simulink model "liner_vs_uliner"  (R2023b)
settings: Solver=VariableStepAuto  StartTime=0.0  StopTime=5  RelTol=1e-9
values from neighbouring files (symbols this model uses):
  A = [A_x, A_y, A_z, A_phi, A_thetha, A_psi]    [Overforingsfunksjon_Translasjon.m]
  Cd = 1.5    [Overforingsfunksjon_Translasjon.m]
  D_jag = [M(1),rho_vann*Cd*A_x*X_2]    [Overforingsfunksjon_Translasjon.m]
  M = M_rb + M_A    [Overforingsfunksjon_Translasjon.m]
  rho_vann = 1000    [Overforingsfunksjon_Translasjon.m]
settings Model: Creator=anneb  LastModifiedBy=anneb

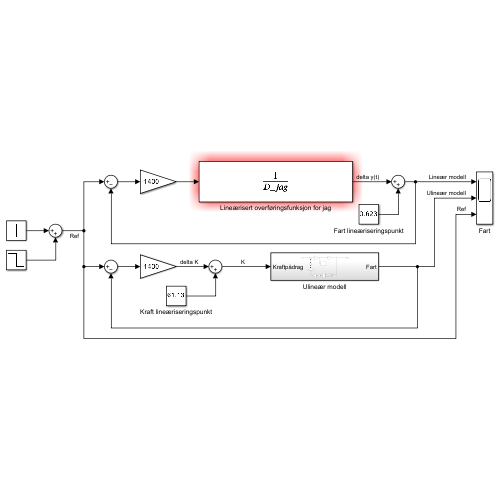
[thumbnail: Simulink's stored preview of the top-level diagram]
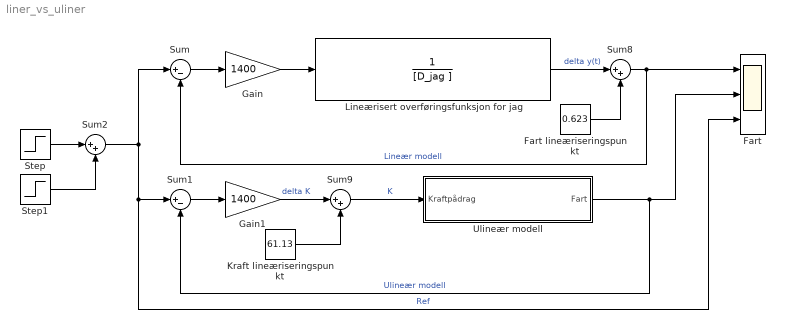
== system liner_vs_uliner ==
  Fart : Scope  NumInputPorts=3
  Fart lineæriseringspunkt : Constant  Value=0.623
  Gain : Gain  Gain=1400
  Gain1 : Gain  Gain=1400
  Kraft lineæriseringspunkt : Constant  Value=61.13
  Lineærisert overføringsfunksjon for jag : TransferFcn  Denominator=[D_jag ]
  Step : Step  Before=0.623  After=0.89  SampleTime=0
  Step1 : Step  Time=3  After=-0.89  SampleTime=0
  Sum : Sum  Inputs=|+-
  Sum1 : Sum  Inputs=|+-
  Sum2 : Sum  Inputs=|++
  Sum8 : Sum  Inputs=|++
  Sum9 : Sum  Inputs=|++
  Ulineær modell : Subsystem
  wires:
  Lineærisert overføringsfunksjon for jag/1 -> Sum8/1  "delta y(t)"
  Sum8/1 -> Sum/2, Fart/1  "Lineær modell"
  Ulineær modell/1(Fart) -> Sum1/2, Fart/2  "Ulineær modell"
  Step/1 -> Sum2/1
  Fart lineæriseringspunkt/1 -> Sum8/2
  Kraft lineæriseringspunkt/1 -> Sum9/2
  Sum9/1 -> Ulineær modell/1(Kraftpådrag)  "K"
  Gain/1 -> Lineærisert overføringsfunksjon for jag/1
  Gain1/1 -> Sum9/1  "delta K"
  Sum/1 -> Gain/1
  Sum1/1 -> Gain1/1
  Step1/1 -> Sum2/2
  Sum2/1 -> Sum1/1, Fart/3, Sum/1  "Ref"

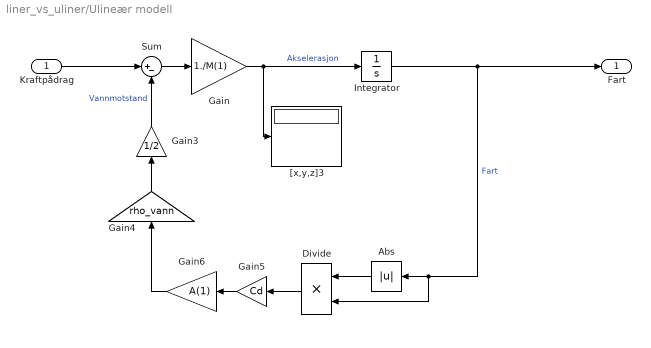
== system liner_vs_uliner/Ulineær modell ==
  Kraftpådrag : Inport
  Abs : Abs  SaturateOnIntegerOverflow=off
  Divide : Product  Inputs=**
  Gain : Gain  Gain=1./M(1)
  Gain3 : Gain  Gain=1/2
  Gain4 : Gain  Gain=rho_vann
  Gain5 : Gain  Gain=Cd
  Gain6 : Gain  Gain=A(1)
  Integrator : Integrator
  Sum : Sum  Inputs=|+-
  "[x,y,z]3" : Display
  Fart : Outport
  wires:
  Gain3/1 -> Sum/2  "Vannmotstand"
  Gain/1 -> "[x,y,z]3"/1, Integrator/1  "Akselerasjon"
  Divide/1 -> Gain5/1
  Gain5/1 -> Gain6/1
  Abs/1 -> Divide/1
  Gain4/1 -> Gain3/1
  Gain6/1 -> Gain4/1
  Sum/1 -> Gain/1
  Integrator/1 -> Abs/1, Divide/2, Fart/1  "Fart"
  Kraftpådrag/1 -> Sum/1
